simulink model "43_BusNetworkElectricityTransmissionModel"  (R2023b)
settings: Solver=VariableStepAuto  StartTime=0.0  StopTime=0.8  RelTol=1e-3
model workspace (MAT data in the model file):
  BESS_Fp_KDroop = 0.025
  BESS_KSI = 817
  BESS_PWM_fs = 560
  BESS_P_Ki = 0.5
  BESS_P_Kp = 0.0636
  BESS_Pnom = 3000000
  BESS_Q_Ki = 1
  BESS_Q_Kp = 0.0257
  BESS_Vd_Ki = 850
  BESS_Vd_Kp = 0.216
  BESS_Vnom = 1000
  BESS_Vq_KDroop = 0.025
  BESS_Vq_Ki = 850
  BESS_Vq_Kp = 0.216
  Compensation_Ki = 30
  Compensation_Kp = 3
  DC_Ki = 400
  DC_Kp = 8
  F = 0.01
  Flux_min = 0.5
  Grid_Freq_PWM = 2700
  Grid_Ireg_Ki = 5
  Grid_Ireg_Kp = 0.83
  Grid_Ireg_lim = 1.1
  Grid_Modindex_Upper = 1.1
  Grid_conv_Imax = 0.8
  H = 0.685
  Idref_max = 0.9
  Iqref_Tc = 0.3
  Ki_Var = 0.05
  Ki_Vreg = 20
  Ksh = 1.1
  L_pu = 0.3
  Llr = 0.16
  Lls = 0.18
  Lm = 2.9
  LowLoad_P = 130
  Nb_wt = 6
  P_mech = 1080000
  PeakShav_P = 200
  Pitch_Ki = 0
  Pitch_Kp = 150
  Pitch_Max = 27
  Pitch_Tc = 0.01
  Pitch_rate = 10
  Q_Filt = 50
  R_pu = 0.003
  Rotor_Freq_PWM = 1620
  Rotor_Ireg_Ki = 8
  Rotor_Ireg_Kp = 0.6
  Rotor_Ireg_lim = 0.1
  Rotor_Modindex_Upper = 2
  Rr = 0.016
  Rs = 0.023
  SOCBESS : Simulink.Parameter (value not decoded)
  T_set = 0.0001
  Tp = 5e-05
  Ts = 5e-06
  Var_C_Filt = 720000
  Var_reg_max = 1.1
  Var_reg_min = 0.9
  WT_Coeff = [0.645 116 0.4 5 21 0.00912 0.08 0.035]
  WT_H = 4.32
  WT_IGBTRon = 5.931
  WT_Param = [91.204 10143]
  Wind_Freq_Filt = 10000
  Wind_Freq_nom = 60
  Wind_P_nom = 1200000
  Wind_Rotor_V_nom = 1950
  Wind_V_nom = 500
  Zeta_Filt = 0.707106781187
  init = [-0.2 0 0 0 0 0 0 0]
  p = 3
  torque0 = 0.83
  v_Ki = 0.1
  v_Kp = 3.6
  v_Max = 1.2
  v_Min = 0.7
  v_T = 5
  vreg_max = 1
  wind_VDC_nom = 1150
  wt0 = 1.2
undefined symbols (not defined in the file): D1, D11, Delta, DiscIntNeverNeededParam, Iabc, Ion, Lithium, P, Q, Vabc
libraries: powerlib_extras x156, spsSeriesRLCBranchLib x66, spsLoadFlowBusLib x43, spsThreePhaseSeriesRLCLoadLib x33, spsThreePhaseTransformerTwoWindingsLib x32, spsThreePhaseVIMeasurementLib x30, simulink_extras x30, spsDistributedParametersLineLib x22, spsGenericPowerSystemStabilizerLib x20, spsSynchronousMachinepuStandardLib x10, spsExcitationSystemLib x10, spsHydraulicTurbineandGovernorLib x10
(part 8 of 19)

== system 43_BusNetworkElectricityTransmissionModel/400 kV Solar Farm/VSC Control/Uabc_ref Generation max (m) = 1 ==
  note: (Correction for transformer
      |  D1 connection)
  note: (Correction for delai of Ts_Control)
  wt : Inport
  VdVq_conv : Inport  Port=2
  Add1 : Sum  Inputs=++++
  Add2 : Sum
  Complex to Magnitude-Angle : ComplexToMagnitudeAngle
  Constant : Constant  Value=-pi/6
  Constant1 : Constant  Value=Vnom_dc
  Constant2 : Constant  Value="[ 0  -2*pi/3  2*pi/3  ]"
  Constant3 : Constant  Value=Vnom_sec*sqrt(2)/sqrt(3)
  Constant4 : Constant  Value=Ts*Fnom*(2*pi)
  Demux1 : Demux  Outputs=2
  Gain1 : Gain  Gain=1/2
  Product : Product  Inputs=*/  RndMeth=Zero
  Product1 : Product  Inputs=*/  RndMeth=Zero
  Product2 : Product  Inputs=**  RndMeth=Zero
  Real-Imag to Complex : RealImagToComplex
  Saturation : Saturate  UpperLimit=1  LowerLimit=0
  Trigonometric Function : Trigonometry
  Uabc_ref : Outport  VectorParamsAs1DForOutWhenUnconnected=off
  wires:
  Complex to Magnitude-Angle/1 -> Saturation/1
  Constant1/1 -> Gain1/1
  VdVq_conv/1 -> Product1/1
  Product1/1 -> Demux1/1
  Gain1/1 -> Product/1
  Real-Imag to Complex/1 -> Complex to Magnitude-Angle/1
  Demux1/1 -> Real-Imag to Complex/1
  Demux1/2 -> Real-Imag to Complex/2
  Constant2/1 -> Add1/2
  Constant/1 -> Add1/3
  Constant3/1 -> Product/2
  Product/1 -> Product1/2
  Complex to Magnitude-Angle/2 -> Add2/1
  Add1/1 -> Add2/2
  Add2/1 -> Trigonometric Function/1
  Saturation/1 -> Product2/1
  Trigonometric Function/1 -> Product2/2
  Product2/1 -> Uabc_ref/1
  wt/1 -> Add1/1
  Constant4/1 -> Add1/4

== system 43_BusNetworkElectricityTransmissionModel/400 kV Solar Farm/VSC Control/VDC Regulator ==
  Vdc_mes : Inport  PortDimensions=1
  Vdc_ref : Inport  Port=2  PortDimensions=1
  PI : slpidlib/PID Controller  Controller=PI  Form=Parallel  TimeDomain=Discrete-time  UseExternalTs=off  SampleTime=Ts  IntegratorMethod=Trapezoidal  FilterMethod=Forward Euler  ControllerParametersSource=internal  P=Kp_VDCreg  I=Ki_VDCreg  UseKiTs=off  D=0  N=100  UseFilter=on  TunerSelectOption=Transfer Function Based (PID Tuner App)  InitialConditionSource=internal  InitialConditionForIntegrator=0  InitialConditionForFilter=0  DifferentiatorICPrevScaledInput=0  ExternalReset=none  TrackingMode=off  Kt=1  LimitOutput=on  SatLimitsSource=internal  UpperSaturationLimit=1.5  LowerSaturationLimit=-1.5  LinearizeAsGain=off  AntiWindupMode=none  Kb=1  LimitIntegrator=off  UpperIntegratorSaturationLimit=inf  LowerIntegratorSaturationLimit=-inf  POutMin=[]  POutMax=[]  IOutMin=[]  IOutMax=[]  DOutMin=[]  DOutMax=[]  NOutMin=[]  NOutMax=[]  SumOutMin=[]  SumOutMax=[]  SaturationOutMin=[]  SaturationOutMax=[]  PParamMin=[]  PParamMax=[]  IParamMin=[]  IParamMax=[]  DParamMin=[]  DParamMax=[]  NParamMin=[]  NParamMax=[]  KbParamMin=[]  KbParamMax=[]  KtParamMin=[]  KtParamMax=[]  KbOutMin=[]  KbOutMax=[]  KtOutMin=[]  KtOutMax=[]  IntegratorOutMin=[]  IntegratorOutMax=[]  FilterOutMin=[]  FilterOutMax=[]  SumI1OutMin=[]  SumI1OutMax=[]  SumI2OutMin=[]  SumI2OutMax=[]  SumI3OutMin=[]  SumI3OutMax=[]  SumI4OutMin=[]  SumI4OutMax=[]  SumDOutMin=[]  SumDOutMax=[]  DifferentiatorOutMin=[]  DifferentiatorOutMax=[]  FilterDiffOutCoefMin=[]  FilterDiffOutCoefMax=[]  ReciprocalOutMin=[]  ReciprocalOutMax=[]  SumDenOutMin=[]  SumDenOutMax=[]  SumNumOutMin=[]  SumNumOutMax=[]  DivideOutMin=[]  DivideOutMax=[]  UdiffTsProdOutMin=[]  UdiffTsProdOutMax=[]  NTsProdOutMin=[]  NTsProdOutMax=[]  UintegralTsProdOutMin=[]  UintegralTsProdOutMax=[]  UngainTsProdOutMin=[]  UngainTsProdOutMax=[]  ClampingZeroOutDataTypeStr=Inherit: Inherit via back propagation  ClampingZeroOutMin=[]  ClampingZeroOutMax=[]  FilterDenConstantOutDataTypeStr=Inherit: Inherit via back propagation  FilterDenConstantOutMin=[]  FilterDenConstantOutMax=[]  PCopyOutDataTypeStr=Inherit: Inherit via back propagation  PCopyOutMin=[]  PCopyOutMax=[]  NCopyOutDataTypeStr=Inherit: Inherit via back propagation  NCopyOutMin=[]  NCopyOutMax=[]  IntegratorContinuousStateAttributes=''  IntegratorStateMustResolveToSignalObject=off  IntegratorRTWStateStorageClass=Auto  FilterContinuousStateAttributes=''  FilterStateMustResolveToSignalObject=off  FilterRTWStateStorageClass=Auto  ParallelPVariant=InternalParameters  IdealPVariant=Disabled  IVariant=InternalParameters  DVariant=Disabled  IntegratorVariant=Discrete  SatVariant=Enabled  AWVariant=Passthrough  PCopyVariant=Disabled  TRVariant=Disabled  FdbkBlocksVariant=Forward  IdealPFdbkVariant=Disabled  SatFdbkVariant=Disabled  DerivativeFilterVariant=Disabled  NVariant=Disabled  NCopyVariant=Disabled_SignalSpec  FilterICVariant=Disabled  IntegratorICVariant=InternalICs  ExternalResetVariant=Disabled  TRSumVariant=Passthrough  SumFdbkVariant=Disabled  SumVariant=Sum_PI  TsampFilterVariant=InternalTs  TsampNgainVariant=Passthrough  TsampIntegralVariant=Disabled_SignalSpec  ExternalSaturationOutDataTypeStr=Inherit: Same as second input
  Rtot_pu3 : Gain  Gain=1/Vnom_dc  SaturateOnIntegerOverflow=on  OutDataTypeStr=Inherit: Same as input  ParamDataTypeStr=Inherit: Same as input
  Sum : Sum  Inputs=|+-
  Id_ref : Outport  SampleTime=Ts  InitialOutput=0  VectorParamsAs1DForOutWhenUnconnected=off
  wires:
  Sum/1 -> Rtot_pu3/1
  Vdc_mes/1 -> Sum/1
  Vdc_ref/1 -> Sum/2
  Rtot_pu3/1 -> PI/1
  PI/1 -> Id_ref/1

== system 43_BusNetworkElectricityTransmissionModel/Li-ion BESS/BESS/BESS and Controller ==
  Control : Inport
  Grid_Data : Inport  Port=2
  BESS : Subsystem
      settings: PortSchema="{\"entries\":[{\"content\":{\"sides\":[{\"content\":{\"connectorIds\":[\"In1\",\"LConn1\",\"LConn2\",\"LConn3\"]},\"type\":\"ConnectorPlacement.EquallySpacedRectSide\",\"uuid\":\"a1d953a5-733c-426a-ade3-c5bdc4580032\"},{\"content\":{\"connectorIds\":[\"In2\",\"Out1\"],\"side\":\"RIGHT\"},\"type\":\"ConnectorPlacement.EquallySpacedRectSide\",\"uuid\":\"97f93640-474b-46b7-9c6f-aa155152508d\"},{\"content\":{\"side\":\"TOP\"},\"type\":\"ConnectorPlacement.EquallySpacedRectSide\",\"uuid\":\"f50f5af6-db0c-4ef7-bd71-a55c9ecceb9a\"}]},\"type\":\"ConnectorPlacement.EquallySpacedConnector\",\"uuid\":\"22d19704-c3d4-4f3f-ab22-c7739cf2dc05\"}],\"packageUris\":[\"http://schema.mathworks.com/mf0/Connector/R2020b\"],\"version\":\"1.0\"}"
  BESS Control : Subsystem
      settings: PortSchema="{\"entries\":[{\"content\":{\"sides\":[{\"content\":{\"connectorIds\":[\"In1\",\"In2\",\"In3\"]},\"type\":\"ConnectorPlacement.EquallySpacedRectSide\",\"uuid\":\"c98aaab3-ca22-4a29-92cf-a6c6fcb60087\"},{\"content\":{\"connectorIds\":[\"Out1\",\"Out2\",\"Out3\"],\"side\":\"RIGHT\"},\"type\":\"ConnectorPlacement.EquallySpacedRectSide\",\"uuid\":\"d7f3f6ce-ab70-4311-9ddf-7d43df8329f4\"},{\"content\":{\"connectorIds\":[\"In4\"],\"side\":\"TOP\"},\"type\":\"ConnectorPlacement.EquallySpacedRectSide\",\"uuid\":\"f981cd0b-01ce-44ec-8804-34a9753b0161\"}]},\"type\":\"ConnectorPlacement.EquallySpacedConnector\",\"uuid\":\"874b0b3a-e878-43a5-a035-a40a954e1edd\"}],\"packageUris\":[\"http://schema.mathworks.com/mf0/Connector/R2020b\"],\"version\":\"1.0\"}"
  BMS : Subsystem
      settings: PortSchema="{\"entries\":[{\"content\":{\"sides\":[{\"content\":{\"connectorIds\":[\"In1\",\"Out2\",\"Out3\"]},\"type\":\"ConnectorPlacement.EquallySpacedRectSide\",\"uuid\":\"90a0640c-776d-46b7-b062-0b224e57e494\"},{\"content\":{\"connectorIds\":[\"Out1\",\"In3\"],\"side\":\"RIGHT\"},\"type\":\"ConnectorPlacement.EquallySpacedRectSide\",\"uuid\":\"dd2d8a9e-5ca6-4aee-a7d3-a7e9cd622cb5\"},{\"content\":{\"connectorIds\":[\"In2\"],\"side\":\"TOP\"},\"type\":\"ConnectorPlacement.EquallySpacedRectSide\",\"uuid\":\"90e91986-9fe4-4870-9173-40c6af706bc8\"}]},\"type\":\"ConnectorPlacement.EquallySpacedConnector\",\"uuid\":\"b96376bb-fdeb-4c13-a438-fbd280210e00\"}],\"packageUris\":[\"http://schema.mathworks.com/mf0/Connector/R2020b\"],\"version\":\"1.0\"}"
  Bus Creator : BusCreator  Inputs=4
  Bus Creator1 : BusCreator  Inputs=2
  Inverter Measurement : Subsystem
  Three-Phase Series RLC Branch : spsThreePhaseSeriesRLCBranchLib/Three-Phase Series RLC Branch  LConnTagsString=A|B|C  RConnTagsString=A|B|C  BranchType=RL  Resistance=1e-1  Inductance=1e-2  Capacitance=1e-6  Measurements=None
  Three-Phase Series RLC Load : spsThreePhaseSeriesRLCLoadLib/Three-Phase Series RLC Load  LConnTagsString=A|B|C  Configuration=Y (grounded)  NominalVoltage=1000  Vabc=[1e3 1e3 1e3]  Vabcp=[1e3 1e3 1e3]  NominalFrequency=60  UnbalancedPower=off  ActivePower=155346  InductivePower=0  CapacitivePower=1e6  Pabc=[10e3 9e3 11e3]  QLabc=[100 90 110]  QCabc=[100 90 110]  Pabcp=[10e3 9e3 11e3]  QLabcp=[100 90 110]  QCabcp=[100 90 110]  Measurements=None  LoadType=constant Z
  Three-Phase Breaker : spsThreePhaseBreakerLib/Three-Phase Breaker  InitialState=open  SwitchA=on  SwitchB=on  SwitchC=on  SwitchTimes="[0  3]"  External=off  BreakerResistance=0.01  SnubberResistance=1e6  SnubberCapacitance=inf  Measurements=None
  A : PMIOPort  Side=Left
  B : PMIOPort  Port=2  Side=Left
  C : PMIOPort  Port=3  Side=Left
  BESS_Data : Outport
  wires:
  Control/1 -> BMS/2(Control), BESS Control/4(Control)
  BMS/2(Stat_BESS) -> Bus Creator/2
  BMS/3(Stat_SOC) -> Bus Creator/3
  Inverter Measurement/1(BESS_Data) -> BESS Control/3(BESS_Data), Bus Creator1/1  "BESS_Data2"
  BESS/1(SOC) -> Bus Creator/4, BMS/3(SOC)  "SoC"
  [BESS_Command] -> Bus Creator/1, BMS/1(BESS_Command)
  Grid_Data/1 -> BESS Control/2(Grid_Data)
  BESS Control/3(BESS_Control) -> Bus Creator1/2  "BMS_Data"
  Bus Creator1/1 -> BESS_Data/1
  BESS Control/2(BMS) -> [BESS_Command]
  BESS Control/1(PWM_Wave) -> BESS/1(PWM wave)
  Bus Creator/1 -> BESS Control/1(BMS_BESS)
  BMS/1(Gate_Op) -> BESS/2(Gate_Op)
  connections:
  Three-Phase Series RLC Branch/RConn3 -- Inverter Measurement/LConn3 -- Three-Phase Series RLC Load/LConn3
  Three-Phase Series RLC Load/LConn1 -- Three-Phase Series RLC Branch/RConn1 -- Inverter Measurement/LConn1
  Three-Phase Series RLC Branch/RConn2 -- Three-Phase Series RLC Load/LConn2 -- Inverter Measurement/LConn2
  Inverter Measurement/RConn1 -- Three-Phase Breaker/LConn1
  Three-Phase Breaker/LConn2 -- Inverter Measurement/RConn2
  Inverter Measurement/RConn3 -- Three-Phase Breaker/LConn3
  Three-Phase Breaker/RConn1 -- A/RConn1
  B/RConn1 -- Three-Phase Breaker/RConn2
  Three-Phase Breaker/RConn3 -- C/RConn1
  BESS/LConn1 -- Three-Phase Series RLC Branch/LConn1
  BESS/LConn2 -- Three-Phase Series RLC Branch/LConn2
  BESS/LConn3 -- Three-Phase Series RLC Branch/LConn3

== system 43_BusNetworkElectricityTransmissionModel/Li-ion BESS/BESS/Grid Measurement ==
  Bus Creator : BusCreator  Inputs=Vabc,Iabc,P,Q
  Power Calculation : Subsystem
  Scope : Scope  NumInputPorts=2
  Three-Phase V-I Measurement : spsThreePhaseVIMeasurementLib/Three-Phase V-I Measurement  VoltageMeasurement=phase-to-ground  SetLabelV=off  LabelV=BESS_Vabc  Vpu=off  VpuLL=off  CurrentMeasurement=yes  SetLabelI=off  LabelI=Iabc  Ipu=off  Pbase=100e6  Vbase=500e3  OutputType=Complex  PhasorSimulation=off  PSBequivalent=0
  A : PMIOPort  Side=Left
  B : PMIOPort  Port=2  Side=Left
  C : PMIOPort  Port=3  Side=Left
  A1 : PMIOPort  Port=4  Side=Right
  B1 : PMIOPort  Port=5  Side=Right
  C1 : PMIOPort  Port=6  Side=Right
  Grid : Outport
  wires:
  Three-Phase V-I Measurement/1 -> Bus Creator/1, Power Calculation/1(Vabc)  "Vabc"
  Three-Phase V-I Measurement/2 -> Bus Creator/2, Power Calculation/2(Iabc)  "Iabc"
  Power Calculation/2(Q) -> Scope/2, Bus Creator/4  "Q"
  Bus Creator/1 -> Grid/1
  Power Calculation/1(P) -> Scope/1, Bus Creator/3  "P"
  connections:
  Three-Phase V-I Measurement/RConn2 -- B1/RConn1
  Three-Phase V-I Measurement/LConn2 -- B/RConn1
  Three-Phase V-I Measurement/LConn3 -- C/RConn1
  C1/RConn1 -- Three-Phase V-I Measurement/RConn3
  A1/RConn1 -- Three-Phase V-I Measurement/RConn1
  A/RConn1 -- Three-Phase V-I Measurement/LConn1

== system 43_BusNetworkElectricityTransmissionModel/Li-ion BESS/Control/Monitoring and measurement  ==
  BESS_Data : Inport
  AND : Logic  IconShape=distinctive  AllPortsSameDT=off  OutDataTypeStr=boolean
  AND1 : Logic  IconShape=distinctive  AllPortsSameDT=off  OutDataTypeStr=boolean
  BESS Measurements : Subsystem
  BESS_Data1 : InportShadow
  BESS_Data3 : InportShadow
  Bus Selector : BusSelector  OutputSignals=Grid_Data.Vabc,Grid_Data.Iabc
  Bus Selector1 : BusSelector  OutputSignals=BESS.BMS_Data.Stat_SOC,BESS.BMS_Data.SoC.MAXSOC,BESS.BMS_Data.SoC.MINSOC,BESS.BMS_Data.signal1.BESS_Charging,BESS.BMS_Data.Stat_BESS,BESS.BMS_Data.signal1.BESS_Discharging
  Bus Selector3 : BusSelector  OutputSignals=BESS.BESS_Data2.P,BESS.BESS_Data2.Q,BESS.BESS_Data2.Vabc,BESS.BESS_Data2.Iabc
  Subsystem : Subsystem
      settings: PortSchema="{\"entries\":[{\"content\":{\"sides\":[{\"content\":{\"connectorIds\":[]},\"type\":\"ConnectorPlacement.EquallySpacedRectSide\",\"uuid\":\"1c641b2f-4abd-4026-9424-76979de06f8f\"},{\"content\":{\"connectorIds\":[\"Out1\"],\"side\":\"RIGHT\"},\"type\":\"ConnectorPlacement.EquallySpacedRectSide\",\"uuid\":\"ecc6cae9-a0ed-4b97-bfc8-2766ee0a977d\"},{\"content\":{\"connectorIds\":[],\"side\":\"TOP\"},\"type\":\"ConnectorPlacement.EquallySpacedRectSide\",\"uuid\":\"9585e64e-ef0f-4765-963d-d981a90f0760\"},{\"content\":{\"connectorIds\":[\"In1\"],\"side\":\"BOTTOM\"},\"type\":\"ConnectorPlacement.EquallySpacedRectSide\",\"uuid\":\"12697e63-83ff-496d-a295-b3930fbd5601\"}]},\"type\":\"ConnectorPlacement.EquallySpacedConnector\",\"uuid\":\"b5fa0ee0-8f2a-44ad-b4f1-35d45efa1097\"}],\"packageUris\":[\"http://schema.mathworks.com/mf0/Connector/R2020b\"],\"version\":\"1.0\"}"
  Subsystem1 : Subsystem
      settings: PortSchema="{\"entries\":[{\"content\":{\"sides\":[{\"content\":{\"connectorIds\":[]},\"type\":\"ConnectorPlacement.EquallySpacedRectSide\",\"uuid\":\"1c641b2f-4abd-4026-9424-76979de06f8f\"},{\"content\":{\"connectorIds\":[\"Out1\"],\"side\":\"RIGHT\"},\"type\":\"ConnectorPlacement.EquallySpacedRectSide\",\"uuid\":\"ecc6cae9-a0ed-4b97-bfc8-2766ee0a977d\"},{\"content\":{\"connectorIds\":[\"In1\"],\"side\":\"TOP\"},\"type\":\"ConnectorPlacement.EquallySpacedRectSide\",\"uuid\":\"9585e64e-ef0f-4765-963d-d981a90f0760\"},{\"content\":{\"connectorIds\":[],\"side\":\"BOTTOM\"},\"type\":\"ConnectorPlacement.EquallySpacedRectSide\",\"uuid\":\"12697e63-83ff-496d-a295-b3930fbd5601\"}]},\"type\":\"ConnectorPlacement.EquallySpacedConnector\",\"uuid\":\"b5fa0ee0-8f2a-44ad-b4f1-35d45efa1097\"}],\"packageUris\":[\"http://schema.mathworks.com/mf0/Connector/R2020b\"],\"version\":\"1.0\"}"
  THD : Scope  NumInputPorts=2
  Total Harmonic Distortion2 : eeTotalHarmonicDistorsion/Total Harmonic Distortion  f=60  Ts=Ts
      settings: LibrarySourceBlock=|
      | ee_sl_lib/Measurements/Total Harmonic
      | Distortion
  Total Harmonic Distortion3 : eeTotalHarmonicDistorsion/Total Harmonic Distortion  f=60  Ts=Ts
      settings: LibrarySourceBlock=|
      | ee_sl_lib/Measurements/Total Harmonic
      | Distortion
  tag scope: BESS_Charge_Actual=global, BESS_Charging_Com=global, BESS_Discharge_Actual=global, BESS_Discharging_Com=global, BESS_MAXSOC=global, BESS_MINSOC=global, BESS_SOC=global, Stat_BESS=global
  wires:
  Bus Selector3/1 -> BESS Measurements/1(BESS_P)  "<P>"
  Bus Selector1/5 -> [Stat_BESS], Subsystem/1(mBESS), Subsystem1/1(mBESS)  "<Stat_BESS>"
  Bus Selector1/6 -> [BESS_Discharging_Com], AND/1  "<BESS_Discharging>"
  Bus Selector1/2 -> [BESS_MAXSOC]  "<MAXSOC>"
  Bus Selector1/3 -> [BESS_MINSOC]  "<MINSOC>"
  Bus Selector1/1 -> [BESS_SOC]  "<Stat_SOC>"
  AND/1 -> [BESS_Discharge_Actual]  "BESS Discharge"
  Bus Selector1/4 -> [BESS_Charging_Com], AND1/2  "<BESS_Charging>"
  AND1/1 -> [BESS_Charge_Actual]  "BESS Charge"
  Subsystem/1(Out1) -> AND/2
  Subsystem1/1(Out1) -> AND1/1
  Total Harmonic Distortion2/1 -> THD/1  "Grid Voltage THD (%)"
  Total Harmonic Distortion3/1 -> THD/2  "Grid Current THD (%)"
  Bus Selector/2 -> Total Harmonic Distortion3/1  "<Iabc>"
  BESS_Data/1 -> Bus Selector/1
  Bus Selector/1 -> Total Harmonic Distortion2/1  "<Vabc>"
  BESS_Data1/1 -> Bus Selector1/1
  BESS_Data3/1 -> Bus Selector3/1
  Bus Selector3/2 -> BESS Measurements/2(BESS_Q)  "<Q>"
  Bus Selector3/3 -> BESS Measurements/3(BESS Voltage)  "<Vabc>"
  Bus Selector3/4 -> BESS Measurements/4(BESS Current)  "<Iabc>"

== system 43_BusNetworkElectricityTransmissionModel/North Network/Regulators 7/Turbine and Excitation Regulators ==
  pref : Inport
  w : Inport  Port=2
  Pe 0 : Inport  Port=3
  Vref : Inport  Port=4
  Vm : Inport  Port=5
  Add : Sum  Inputs=+-
  Complex to Real-Imag : ComplexToRealImag
  Excitation System : spsExcitationSystemLib/Excitation System  tr=20e-3  reg=[ 300, 0.001 ]  exc=[ 1, 0 ]  tgr=[ 0, 0 ]  damp=[ 0.001, 0.1 ]  sat=[ 0, 0 ]  lim=[ -11.5, 11.5, 0 ]  v0="[1.0  1.28]"
      settings: LibrarySourceBlock=sps_lib/Electrical Machines/Synchronous Machine Control/Excitation System
  Hydraulic Turbine and Governor : spsHydraulicTurbineandGovernorLib/Hydraulic Turbine and Governor  sm="[ 10/3  0.07 ]"  gate="[  0.01  0.97518  -0.1  0.1 ]"  reg="[  0.05  1.163  0.105  0  0.01  ]"  hyd="[  0  2.67  ]"  dref=0  po=0.7516
      settings: LibrarySourceBlock=|
      | sps_lib/Electrical Machines/Synchronous Machine Control/Hydraulic Turbine
      | and Governor
  Stabilitator : Subsystem
  Terminator : Terminator
  wref : Constant
  wref1 : Constant
  Pm : Outport
  Vf : Outport  Port=2
  wires:
  pref/1 -> Hydraulic Turbine and Governor/2
  Complex to Real-Imag/2 -> Excitation System/3
  wref/1 -> Hydraulic Turbine and Governor/1
  Add/1 -> Stabilitator/3(dw), Hydraulic Turbine and Governor/5
  Vm/1 -> Complex to Real-Imag/1
  Pe 0/1 -> Stabilitator/2(Pe), Hydraulic Turbine and Governor/4
  Hydraulic Turbine and Governor/2 -> Terminator/1
  Stabilitator/1(Out1) -> Excitation System/4
  w/1 -> Add/1, Hydraulic Turbine and Governor/3
  Excitation System/1 -> Vf/1
  Hydraulic Turbine and Governor/1 -> Pm/1, Stabilitator/1(Pm)
  Vref/1 -> Excitation System/1
  wref1/1 -> Add/2
  Complex to Real-Imag/1 -> Excitation System/2

== system 43_BusNetworkElectricityTransmissionModel/North Network/Regulators 8/Turbine and Excitation Regulators ==
  pref : Inport
  w : Inport  Port=2
  Pe 0 : Inport  Port=3
  Vref : Inport  Port=4
  Vm : Inport  Port=5
  Add : Sum  Inputs=+-
  Complex to Real-Imag : ComplexToRealImag
  Excitation System : spsExcitationSystemLib/Excitation System  tr=20e-3  reg=[ 300, 0.001 ]  exc=[ 1, 0 ]  tgr=[ 0, 0 ]  damp=[ 0.001, 0.1 ]  sat=[ 0, 0 ]  lim=[ -11.5, 11.5, 0 ]  v0="[1.0  1.28]"
      settings: LibrarySourceBlock=sps_lib/Electrical Machines/Synchronous Machine Control/Excitation System
  Hydraulic Turbine and Governor : spsHydraulicTurbineandGovernorLib/Hydraulic Turbine and Governor  sm="[ 10/3  0.07 ]"  gate="[  0.01  0.97518  -0.1  0.1 ]"  reg="[  0.05  1.163  0.105  0  0.01  ]"  hyd="[  0  2.67  ]"  dref=0  po=0.7516
      settings: LibrarySourceBlock=|
      | sps_lib/Electrical Machines/Synchronous Machine Control/Hydraulic Turbine
      | and Governor
  Stabilitator : Subsystem
  Terminator : Terminator
  wref : Constant
  wref1 : Constant
  Pm : Outport
  Vf : Outport  Port=2
  wires:
  pref/1 -> Hydraulic Turbine and Governor/2
  Complex to Real-Imag/2 -> Excitation System/3
  wref/1 -> Hydraulic Turbine and Governor/1
  Add/1 -> Stabilitator/3(dw), Hydraulic Turbine and Governor/5
  Vm/1 -> Complex to Real-Imag/1
  Pe 0/1 -> Stabilitator/2(Pe), Hydraulic Turbine and Governor/4
  Hydraulic Turbine and Governor/2 -> Terminator/1
  Stabilitator/1(Out1) -> Excitation System/4
  w/1 -> Add/1, Hydraulic Turbine and Governor/3
  Excitation System/1 -> Vf/1
  Hydraulic Turbine and Governor/1 -> Pm/1, Stabilitator/1(Pm)
  Vref/1 -> Excitation System/1
  wref1/1 -> Add/2
  Complex to Real-Imag/1 -> Excitation System/2

== system 43_BusNetworkElectricityTransmissionModel/North Network/Regulators 9/Turbine and Excitation Regulators ==
  pref : Inport
  w : Inport  Port=2
  Pe 0 : Inport  Port=3
  Vref : Inport  Port=4
  Vm : Inport  Port=5
  Add : Sum  Inputs=+-
  Complex to Real-Imag : ComplexToRealImag
  Excitation System : spsExcitationSystemLib/Excitation System  tr=20e-3  reg=[ 300, 0.001 ]  exc=[ 1, 0 ]  tgr=[ 0, 0 ]  damp=[ 0.001, 0.1 ]  sat=[ 0, 0 ]  lim=[ -11.5, 11.5, 0 ]  v0="[1.0  1.28]"
      settings: LibrarySourceBlock=sps_lib/Electrical Machines/Synchronous Machine Control/Excitation System
  Hydraulic Turbine and Governor : spsHydraulicTurbineandGovernorLib/Hydraulic Turbine and Governor  sm="[ 10/3  0.07 ]"  gate="[  0.01  0.97518  -0.1  0.1 ]"  reg="[  0.05  1.163  0.105  0  0.01  ]"  hyd="[  0  2.67  ]"  dref=0  po=0.7516
      settings: LibrarySourceBlock=|
      | sps_lib/Electrical Machines/Synchronous Machine Control/Hydraulic Turbine
      | and Governor
  Stabilitator : Subsystem
  Terminator : Terminator
  wref : Constant
  wref1 : Constant
  Pm : Outport
  Vf : Outport  Port=2
  wires:
  pref/1 -> Hydraulic Turbine and Governor/2
  Complex to Real-Imag/2 -> Excitation System/3
  wref/1 -> Hydraulic Turbine and Governor/1
  Add/1 -> Stabilitator/3(dw), Hydraulic Turbine and Governor/5
  Vm/1 -> Complex to Real-Imag/1
  Pe 0/1 -> Stabilitator/2(Pe), Hydraulic Turbine and Governor/4
  Hydraulic Turbine and Governor/2 -> Terminator/1
  Stabilitator/1(Stab) -> Excitation System/4
  w/1 -> Add/1, Hydraulic Turbine and Governor/3
  Excitation System/1 -> Vf/1
  Hydraulic Turbine and Governor/1 -> Pm/1, Stabilitator/1(Pm)
  Vref/1 -> Excitation System/1
  wref1/1 -> Add/2
  Complex to Real-Imag/1 -> Excitation System/2

== system 43_BusNetworkElectricityTransmissionModel/Regulators 10/Turbine and Excitation Regulators/Stabilitator ==
  Pm : Inport
  Pe : Inport  Port=2
  dw : Inport  Port=3
  Add1 : Sum  Inputs=+-
  Generic Power System Stabilizer : spsGenericPowerSystemStabilizerLib/Generic Power System Stabilizer  Tsensor=30e-3  K=20  Twashout=2  Tleadlag1=[50e-3 20e-3]  Tleadlag2=[3 5.4]  VSlimits=[-0.15 0.15]  Vinit=0  Plot_On=off  MagdB_On=on  FreqRange=logspace(-2,2,500)
      settings: LibrarySourceBlock=|
      | sps_lib/Electrical Machines/Synchronous Machine Control/Generic
      | Power System Stabilizer
  Generic Power System Stabilizer1 : spsGenericPowerSystemStabilizerLib/Generic Power System Stabilizer  Tsensor=30e-3  K=20  Twashout=2  Tleadlag1=[50e-3 20e-3]  Tleadlag2=[3 5.4]  VSlimits=[-0.15 0.15]  Vinit=0  Plot_On=off  MagdB_On=on  FreqRange=logspace(-2,2,500)
      settings: LibrarySourceBlock=|
      | sps_lib/Electrical Machines/Synchronous Machine Control/Generic
      | Power System Stabilizer
  Ground : Ground
  Multiport Switch : MultiPortSwitch  DiagnosticForDefault=None  SaturateOnIntegerOverflow=off  InputSameDT=off
  Out1 : Outport
  wires:
  Pm/1 -> Add1/1
  Generic Power System Stabilizer1/1 -> Multiport Switch/4
  Pe/1 -> Add1/2
  Add1/1 -> Generic Power System Stabilizer/1
  Generic Power System Stabilizer/1 -> Multiport Switch/3
  dw/1 -> Generic Power System Stabilizer1/1
  Ground/1 -> Multiport Switch/2
  [PSS_modes] -> Multiport Switch/1
  Multiport Switch/1 -> Out1/1

== system 43_BusNetworkElectricityTransmissionModel/South Network/Regulators 1/Turbine and Excitation Regulators ==
  pref : Inport
  w : Inport  Port=2
  Pe 0 : Inport  Port=3
  Vref : Inport  Port=4
  Vm : Inport  Port=5
  Add : Sum  Inputs=+-
  Complex to Real-Imag : ComplexToRealImag
  Excitation System : spsExcitationSystemLib/Excitation System  tr=20e-3  reg=[ 300, 0.001 ]  exc=[ 1, 0 ]  tgr=[ 0, 0 ]  damp=[ 0.001, 0.1 ]  sat=[ 0, 0 ]  lim=[ -11.5, 11.5, 0 ]  v0="[1.0  1.28]"
      settings: LibrarySourceBlock=sps_lib/Electrical Machines/Synchronous Machine Control/Excitation System
  Hydraulic Turbine and Governor : spsHydraulicTurbineandGovernorLib/Hydraulic Turbine and Governor  sm="[ 10/3  0.07 ]"  gate="[  0.01  0.97518  -0.1  0.1 ]"  reg="[  0.05  1.163  0.105  0  0.01  ]"  hyd="[  0  2.67  ]"  dref=0  po=0.7516
      settings: LibrarySourceBlock=|
      | sps_lib/Electrical Machines/Synchronous Machine Control/Hydraulic Turbine
      | and Governor
  Stabilitator : Subsystem
  Terminator : Terminator
  wref : Constant
  wref1 : Constant
  Pm : Outport
  Vf : Outport  Port=2
  wires:
  pref/1 -> Hydraulic Turbine and Governor/2
  Complex to Real-Imag/2 -> Excitation System/3
  wref/1 -> Hydraulic Turbine and Governor/1
  Add/1 -> Stabilitator/3(dw), Hydraulic Turbine and Governor/5
  Vm/1 -> Complex to Real-Imag/1
  Pe 0/1 -> Stabilitator/2(Pe), Hydraulic Turbine and Governor/4
  Hydraulic Turbine and Governor/2 -> Terminator/1
  Stabilitator/1(Out1) -> Excitation System/4
  w/1 -> Add/1, Hydraulic Turbine and Governor/3
  Excitation System/1 -> Vf/1
  Hydraulic Turbine and Governor/1 -> Pm/1, Stabilitator/1(Pm)
  Vref/1 -> Excitation System/1
  wref1/1 -> Add/2
  Complex to Real-Imag/1 -> Excitation System/2

== system 43_BusNetworkElectricityTransmissionModel/South Network/Regulators 2/Turbine and Excitation Regulators ==
  pref : Inport
  w : Inport  Port=2
  Pe 0 : Inport  Port=3
  Vref : Inport  Port=4
  Vm : Inport  Port=5
  Add : Sum  Inputs=+-
  Complex to Real-Imag : ComplexToRealImag
  Excitation System : spsExcitationSystemLib/Excitation System  tr=20e-3  reg=[ 300, 0.001 ]  exc=[ 1, 0 ]  tgr=[ 0, 0 ]  damp=[ 0.001, 0.1 ]  sat=[ 0, 0 ]  lim=[ -11.5, 11.5, 0 ]  v0="[1.0  1.28]"
      settings: LibrarySourceBlock=sps_lib/Electrical Machines/Synchronous Machine Control/Excitation System
  Hydraulic Turbine and Governor : spsHydraulicTurbineandGovernorLib/Hydraulic Turbine and Governor  sm="[ 10/3  0.07 ]"  gate="[  0.01  0.97518  -0.1  0.1 ]"  reg="[  0.05  1.163  0.105  0  0.01  ]"  hyd="[  0  2.67  ]"  dref=0  po=0.7516
      settings: LibrarySourceBlock=|
      | sps_lib/Electrical Machines/Synchronous Machine Control/Hydraulic Turbine
      | and Governor
  Stabilitator : Subsystem
  Terminator : Terminator
  wref : Constant
  wref1 : Constant
  Pm : Outport
  Vf : Outport  Port=2
  wires:
  pref/1 -> Hydraulic Turbine and Governor/2
  Complex to Real-Imag/2 -> Excitation System/3
  wref/1 -> Hydraulic Turbine and Governor/1
  Add/1 -> Stabilitator/3(dw), Hydraulic Turbine and Governor/5
  Vm/1 -> Complex to Real-Imag/1
  Pe 0/1 -> Stabilitator/2(Pe), Hydraulic Turbine and Governor/4
  Hydraulic Turbine and Governor/2 -> Terminator/1
  Stabilitator/1(Out1) -> Excitation System/4
  w/1 -> Add/1, Hydraulic Turbine and Governor/3
  Excitation System/1 -> Vf/1
  Hydraulic Turbine and Governor/1 -> Pm/1, Stabilitator/1(Pm)
  Vref/1 -> Excitation System/1
  wref1/1 -> Add/2
  Complex to Real-Imag/1 -> Excitation System/2

== system 43_BusNetworkElectricityTransmissionModel/South Network/Regulators 3/Turbine and Excitation Regulators ==
  pref : Inport
  w : Inport  Port=2
  Pe 0 : Inport  Port=3
  Vref : Inport  Port=4
  Vm : Inport  Port=5
  Add : Sum  Inputs=+-
  Complex to Real-Imag : ComplexToRealImag
  Excitation System : spsExcitationSystemLib/Excitation System  tr=20e-3  reg=[ 300, 0.001 ]  exc=[ 1, 0 ]  tgr=[ 0, 0 ]  damp=[ 0.001, 0.1 ]  sat=[ 0, 0 ]  lim=[ -11.5, 11.5, 0 ]  v0="[1.0  1.28]"
      settings: LibrarySourceBlock=sps_lib/Electrical Machines/Synchronous Machine Control/Excitation System
  Hydraulic Turbine and Governor : spsHydraulicTurbineandGovernorLib/Hydraulic Turbine and Governor  sm="[ 10/3  0.07 ]"  gate="[  0.01  0.97518  -0.1  0.1 ]"  reg="[  0.05  1.163  0.105  0  0.01  ]"  hyd="[  0  2.67  ]"  dref=0  po=0.7516
      settings: LibrarySourceBlock=|
      | sps_lib/Electrical Machines/Synchronous Machine Control/Hydraulic Turbine
      | and Governor
  Stabilitator : Subsystem
  Terminator : Terminator
  wref : Constant
  wref1 : Constant
  Pm : Outport
  Vf : Outport  Port=2
  wires:
  pref/1 -> Hydraulic Turbine and Governor/2
  Complex to Real-Imag/2 -> Excitation System/3
  wref/1 -> Hydraulic Turbine and Governor/1
  Add/1 -> Stabilitator/3(dw), Hydraulic Turbine and Governor/5
  Vm/1 -> Complex to Real-Imag/1
  Pe 0/1 -> Stabilitator/2(Pe), Hydraulic Turbine and Governor/4
  Hydraulic Turbine and Governor/2 -> Terminator/1
  Stabilitator/1(Out1) -> Excitation System/4
  w/1 -> Add/1, Hydraulic Turbine and Governor/3
  Excitation System/1 -> Vf/1
  Hydraulic Turbine and Governor/1 -> Pm/1, Stabilitator/1(Pm)
  Vref/1 -> Excitation System/1
  wref1/1 -> Add/2
  Complex to Real-Imag/1 -> Excitation System/2

== system 43_BusNetworkElectricityTransmissionModel/South Network/Regulators 4/Turbine and Excitation Regulators ==
  pref : Inport
  w : Inport  Port=2
  Pe 0 : Inport  Port=3
  Vref : Inport  Port=4
  Vm : Inport  Port=5
  Add : Sum  Inputs=+-
  Complex to Real-Imag : ComplexToRealImag
  Excitation System : spsExcitationSystemLib/Excitation System  tr=20e-3  reg=[ 300, 0.001 ]  exc=[ 1, 0 ]  tgr=[ 0, 0 ]  damp=[ 0.001, 0.1 ]  sat=[ 0, 0 ]  lim=[ -11.5, 11.5, 0 ]  v0="[1.0  1.28]"
      settings: LibrarySourceBlock=sps_lib/Electrical Machines/Synchronous Machine Control/Excitation System
  Hydraulic Turbine and Governor : spsHydraulicTurbineandGovernorLib/Hydraulic Turbine and Governor  sm="[ 10/3  0.07 ]"  gate="[  0.01  0.97518  -0.1  0.1 ]"  reg="[  0.05  1.163  0.105  0  0.01  ]"  hyd="[  0  2.67  ]"  dref=0  po=0.7516
      settings: LibrarySourceBlock=|
      | sps_lib/Electrical Machines/Synchronous Machine Control/Hydraulic Turbine
      | and Governor
  Stabilitator : Subsystem
  Terminator : Terminator
  wref : Constant
  wref1 : Constant
  Pm : Outport
  Vf : Outport  Port=2
  wires:
  pref/1 -> Hydraulic Turbine and Governor/2
  Complex to Real-Imag/2 -> Excitation System/3
  wref/1 -> Hydraulic Turbine and Governor/1
  Add/1 -> Hydraulic Turbine and Governor/5, Stabilitator/3(dw)
  Vm/1 -> Complex to Real-Imag/1
  Pe 0/1 -> Stabilitator/2(Pe), Hydraulic Turbine and Governor/4
  Hydraulic Turbine and Governor/2 -> Terminator/1
  Stabilitator/1(Out1) -> Excitation System/4
  w/1 -> Add/1, Hydraulic Turbine and Governor/3
  Excitation System/1 -> Vf/1
  Hydraulic Turbine and Governor/1 -> Pm/1, Stabilitator/1(Pm)
  Vref/1 -> Excitation System/1
  wref1/1 -> Add/2
  Complex to Real-Imag/1 -> Excitation System/2

== system 43_BusNetworkElectricityTransmissionModel/South Network/Regulators 5/Turbine and Excitation Regulators ==
  pref : Inport
  w : Inport  Port=2
  Pe 0 : Inport  Port=3
  Vref : Inport  Port=4
  Vm : Inport  Port=5
  Add : Sum  Inputs=+-
  Complex to Real-Imag : ComplexToRealImag
  Excitation System : spsExcitationSystemLib/Excitation System  tr=20e-3  reg=[ 300, 0.001 ]  exc=[ 1, 0 ]  tgr=[ 0, 0 ]  damp=[ 0.001, 0.1 ]  sat=[ 0, 0 ]  lim=[ -11.5, 11.5, 0 ]  v0="[1.0  1.28]"
      settings: LibrarySourceBlock=sps_lib/Electrical Machines/Synchronous Machine Control/Excitation System
  Hydraulic Turbine and Governor : spsHydraulicTurbineandGovernorLib/Hydraulic Turbine and Governor  sm="[ 10/3  0.07 ]"  gate="[  0.01  0.97518  -0.1  0.1 ]"  reg="[  0.05  1.163  0.105  0  0.01  ]"  hyd="[  0  2.67  ]"  dref=0  po=0.7516
      settings: LibrarySourceBlock=|
      | sps_lib/Electrical Machines/Synchronous Machine Control/Hydraulic Turbine
      | and Governor
  Stabilitator : Subsystem
  Terminator : Terminator
  wref : Constant
  wref1 : Constant
  Pm : Outport
  Vf : Outport  Port=2
  wires:
  pref/1 -> Hydraulic Turbine and Governor/2
  Complex to Real-Imag/2 -> Excitation System/3
  wref/1 -> Hydraulic Turbine and Governor/1
  Add/1 -> Stabilitator/3(dw), Hydraulic Turbine and Governor/5
  Vm/1 -> Complex to Real-Imag/1
  Pe 0/1 -> Stabilitator/2(Pe), Hydraulic Turbine and Governor/4
  Hydraulic Turbine and Governor/2 -> Terminator/1
  Stabilitator/1(Out1) -> Excitation System/4
  w/1 -> Add/1, Hydraulic Turbine and Governor/3
  Excitation System/1 -> Vf/1
  Hydraulic Turbine and Governor/1 -> Pm/1, Stabilitator/1(Pm)
  Vref/1 -> Excitation System/1
  wref1/1 -> Add/2
  Complex to Real-Imag/1 -> Excitation System/2

== system 43_BusNetworkElectricityTransmissionModel/South Network/Regulators 6/Turbine and Excitation Regulators ==
  pref : Inport
  w : Inport  Port=2
  Pe 0 : Inport  Port=3
  Vref : Inport  Port=4
  Vm : Inport  Port=5
  Add : Sum  Inputs=+-
  Complex to Real-Imag : ComplexToRealImag
  Excitation System : spsExcitationSystemLib/Excitation System  tr=20e-3  reg=[ 300, 0.001 ]  exc=[ 1, 0 ]  tgr=[ 0, 0 ]  damp=[ 0.001, 0.1 ]  sat=[ 0, 0 ]  lim=[ -11.5, 11.5, 0 ]  v0="[1.0  1.28]"
      settings: LibrarySourceBlock=sps_lib/Electrical Machines/Synchronous Machine Control/Excitation System
  Hydraulic Turbine and Governor : spsHydraulicTurbineandGovernorLib/Hydraulic Turbine and Governor  sm="[ 10/3  0.07 ]"  gate="[  0.01  0.97518  -0.1  0.1 ]"  reg="[  0.05  1.163  0.105  0  0.01  ]"  hyd="[  0  2.67  ]"  dref=0  po=0.7516
      settings: LibrarySourceBlock=|
      | sps_lib/Electrical Machines/Synchronous Machine Control/Hydraulic Turbine
      | and Governor
  Stabilitator : Subsystem
  Terminator : Terminator
  wref : Constant
  wref1 : Constant
  Pm : Outport
  Vf : Outport  Port=2
  wires:
  pref/1 -> Hydraulic Turbine and Governor/2
  Complex to Real-Imag/2 -> Excitation System/3
  wref/1 -> Hydraulic Turbine and Governor/1
  Add/1 -> Stabilitator/3(dw), Hydraulic Turbine and Governor/5
  Vm/1 -> Complex to Real-Imag/1
  Pe 0/1 -> Stabilitator/2(Pe), Hydraulic Turbine and Governor/4
  Hydraulic Turbine and Governor/2 -> Terminator/1
  Stabilitator/1(Out1) -> Excitation System/4
  w/1 -> Add/1, Hydraulic Turbine and Governor/3
  Excitation System/1 -> Vf/1
  Hydraulic Turbine and Governor/1 -> Pm/1, Stabilitator/1(Pm)
  Vref/1 -> Excitation System/1
  wref1/1 -> Add/2
  Complex to Real-Imag/1 -> Excitation System/2

== system 43_BusNetworkElectricityTransmissionModel/ 41.4 MW Wind Generation/41.4 MW Wind Farm/10.35 MW Wind Turbine 1/Wind Turbine & Generator 1 ==
  Generator speed (pu) : Inport
  Constant : Constant  Value=14
  Shaft : Subsystem
  Turbine : Subsystem
  "Wind Turbine " : Subsystem  mask{WT_Coeff8=WT_Coeff, WT_Param=WT_Param, vw0=11, Pmech_Out=1.035e7, Ts=Ts}
      mask prompts: WT_Coeff8 "Wind Turbine Coefficients"; WT_Param "Wind Turbine Coefficients"; vw0 "Initial Wind Speed (m/s)"; Pmech_Out "Nominal Mechanical Output Power"; Ts "Sample Time"
  T_shaft (pu) : Outport  VectorParamsAs1DForOutWhenUnconnected=off
  wires:
  [Pitch_WT1] -> "Wind Turbine "/2(Pitch angle (deg))
  Shaft/1(T_shaft (pu)) -> T_shaft (pu)/1, Turbine/2(T_shaft (pu))
  Generator speed (pu)/1 -> Turbine/3(Generator speed (pu))
  Turbine/2(W_wt (pu)) -> "Wind Turbine "/1(Generator speed (pu)1)
  Turbine/1(Turbine speed) -> Shaft/1(Speed)
  Constant/1 -> "Wind Turbine "/3(Wind speed (m/s))
  "Wind Turbine "/1(Tt (pu)) -> Turbine/1(T_wt (pu))

== system 43_BusNetworkElectricityTransmissionModel/ 41.4 MW Wind Generation/41.4 MW Wind Farm/10.35 MW Wind Turbine 2/Wind Turbine & Generator 1 ==
  Generator speed (pu) : Inport
  Constant : Constant  Value=14
  Shaft : Subsystem
  Turbine : Subsystem
  "Wind Turbine " : Subsystem  mask{WT_Coeff8=WT_Coeff, WT_Param=WT_Param, vw0=11, Pmech_Out=1.035e7, Ts=Ts}
      mask prompts: WT_Coeff8 "Wind Turbine Coefficients"; WT_Param "Wind Turbine Coefficients"; vw0 "Initial Wind Speed (m/s)"; Pmech_Out "Nominal Mechanical Output Power"; Ts "Sample Time"
  T_shaft (pu) : Outport  VectorParamsAs1DForOutWhenUnconnected=off
  wires:
  [Pitch_WT1] -> "Wind Turbine "/2(Pitch angle (deg))
  Shaft/1(T_shaft (pu)) -> T_shaft (pu)/1, Turbine/2(T_shaft (pu))
  Generator speed (pu)/1 -> Turbine/3(Generator speed (pu))
  Turbine/2(W_wt (pu)) -> "Wind Turbine "/1(Generator speed (pu)1)
  Turbine/1(Turbine speed) -> Shaft/1(Speed)
  Constant/1 -> "Wind Turbine "/3(Wind speed (m/s))
  "Wind Turbine "/1(Tt (pu)) -> Turbine/1(T_wt (pu))

== system 43_BusNetworkElectricityTransmissionModel/ 41.4 MW Wind Generation/41.4 MW Wind Farm/10.35 MW Wind Turbine 3/Wind Turbine & Generator 1 ==
  Generator speed (pu) : Inport
  Constant : Constant  Value=14
  Shaft : Subsystem
  Turbine : Subsystem
  "Wind Turbine " : Subsystem  mask{WT_Coeff8=WT_Coeff, WT_Param=WT_Param, vw0=11, Pmech_Out=1.035e7, Ts=Ts}
      mask prompts: WT_Coeff8 "Wind Turbine Coefficients"; WT_Param "Wind Turbine Coefficients"; vw0 "Initial Wind Speed (m/s)"; Pmech_Out "Nominal Mechanical Output Power"; Ts "Sample Time"
  T_shaft (pu) : Outport  VectorParamsAs1DForOutWhenUnconnected=off
  wires:
  [Pitch_WT1] -> "Wind Turbine "/2(Pitch angle (deg))
  Shaft/1(T_shaft (pu)) -> T_shaft (pu)/1, Turbine/2(T_shaft (pu))
  Generator speed (pu)/1 -> Turbine/3(Generator speed (pu))
  Turbine/2(W_wt (pu)) -> "Wind Turbine "/1(Generator speed (pu)1)
  Turbine/1(Turbine speed) -> Shaft/1(Speed)
  Constant/1 -> "Wind Turbine "/3(Wind speed (m/s))
  "Wind Turbine "/1(Tt (pu)) -> Turbine/1(T_wt (pu))

== system 43_BusNetworkElectricityTransmissionModel/ 41.4 MW Wind Generation/41.4 MW Wind Farm/10.35 MW Wind Turbine 4/Wind Turbine & Generator 1 ==
  Generator speed (pu) : Inport
  Constant : Constant  Value=14
  Shaft : Subsystem
  Turbine : Subsystem
  "Wind Turbine " : Subsystem  mask{WT_Coeff8=WT_Coeff, WT_Param=WT_Param, vw0=11, Pmech_Out=1.035e7, Ts=Ts}
      mask prompts: WT_Coeff8 "Wind Turbine Coefficients"; WT_Param "Wind Turbine Coefficients"; vw0 "Initial Wind Speed (m/s)"; Pmech_Out "Nominal Mechanical Output Power"; Ts "Sample Time"
  T_shaft (pu) : Outport  VectorParamsAs1DForOutWhenUnconnected=off
  wires:
  [Pitch_WT1] -> "Wind Turbine "/2(Pitch angle (deg))
  Shaft/1(T_shaft (pu)) -> T_shaft (pu)/1, Turbine/2(T_shaft (pu))
  Generator speed (pu)/1 -> Turbine/3(Generator speed (pu))
  Turbine/2(W_wt (pu)) -> "Wind Turbine "/1(Generator speed (pu)1)
  Turbine/1(Turbine speed) -> Shaft/1(Speed)
  Constant/1 -> "Wind Turbine "/3(Wind speed (m/s))
  "Wind Turbine "/1(Tt (pu)) -> Turbine/1(T_wt (pu))

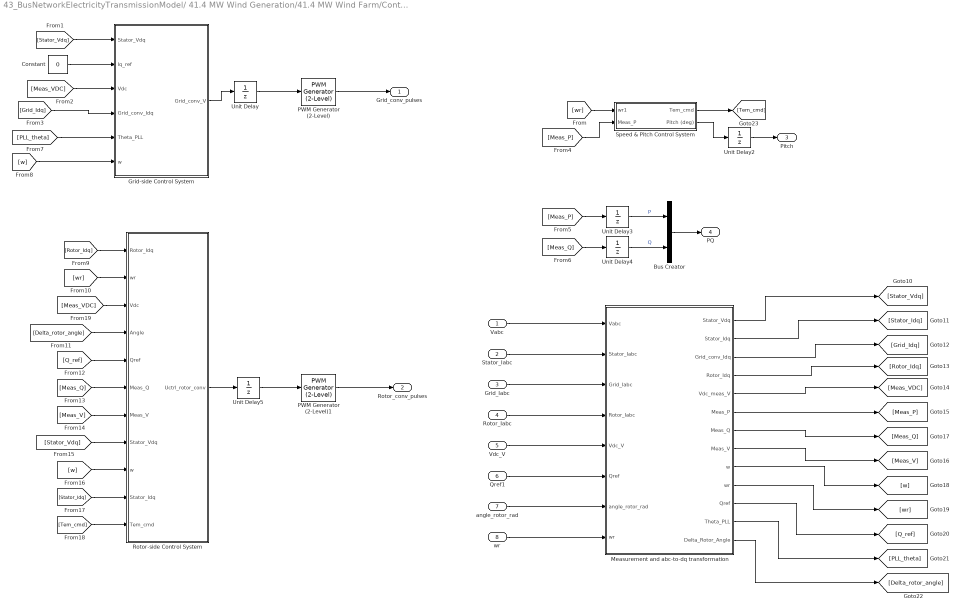
== system 43_BusNetworkElectricityTransmissionModel/ 41.4 MW Wind Generation/41.4 MW Wind Farm/Control System/Control System 1 ==
  Vabc : Inport
  Stator_Iabc : Inport  Port=2
  Grid_Iabc : Inport  Port=3
  Rotor_Iabc : Inport  Port=4
  Vdc_V : Inport  Port=5
  Qref1 : Inport  Port=6
  angle_rotor_rad : Inport  Port=7
  wr : Inport  Port=8
  Bus Creator : BusCreator  Inputs=P,Q
  Constant : Constant  Value=0
  Grid-side Control System : Subsystem
  "Measurement and abc-to-dq transformation " : Subsystem
  PWM Generator (2-Level) : spsPWMGenerator2LevelLib/PWM Generator (2-Level)  ModulatorType=Three-phase bridge (6 pulses)  ModulatorMode=Unsynchronized  Fc=Grid_Freq_PWM  Pc=90  nF=27  MinMax="[ -1  1 ]"  SamplingTechnique=Natural  ModulatingSignals=off  m=0.8  Freq=60  Phase=0  Ts=Ts  ShowCarrierOutport=off
  PWM Generator (2-Level)1 : spsPWMGenerator2LevelLib/PWM Generator (2-Level)  ModulatorType=Three-phase bridge (6 pulses)  ModulatorMode=Unsynchronized  Fc=Rotor_Freq_PWM  Pc=90  nF=27  MinMax="[ -1  1 ]"  SamplingTechnique=Natural  ModulatingSignals=off  m=0.8  Freq=60  Phase=0  Ts=Ts  ShowCarrierOutport=off
  Rotor-side Control System : Subsystem
  Speed & Pitch Control System : Subsystem
  Unit Delay{,2..5} (5 alike) : UnitDelay  SampleTime=Ts  HasFrameUpgradeWarning=on
  Grid_conv_pulses : Outport
  Rotor_conv_pulses : Outport  Port=2
  Pitch : Outport  Port=3
  PQ : Outport  Port=4
  wires:
  [Meas_P] -> Speed & Pitch Control System/2(Meas_P)
  "Measurement and abc-to-dq transformation "/1(Stator_Vdq) -> [Stator_Vdq]
  [Meas_Q] -> Unit Delay4/1
  Unit Delay4/1 -> Bus Creator/2  "Q"
  "Measurement and abc-to-dq transformation "/2(Stator_Idq) -> [Stator_Idq]
  "Measurement and abc-to-dq transformation "/9(w) -> [w]
  Grid_Iabc/1 -> "Measurement and abc-to-dq transformation "/3(Grid_Iabc)
  Grid-side Control System/1(Grid_conv_V) -> Unit Delay/1
  Unit Delay5/1 -> PWM Generator (2-Level)1/1
  Unit Delay2/1 -> Pitch/1
  Unit Delay/1 -> PWM Generator (2-Level)/1
  "Measurement and abc-to-dq transformation "/3(Grid_conv_Idq) -> [Grid_Idq]
  Rotor-side Control System/1(Uctrl_rotor_conv) -> Unit Delay5/1
  "Measurement and abc-to-dq transformation "/13(Delta_Rotor_Angle) -> [Delta_rotor_angle]
  PWM Generator (2-Level)/1 -> Grid_conv_pulses/1
  Vabc/1 -> "Measurement and abc-to-dq transformation "/1(Vabc)
  PWM Generator (2-Level)1/1 -> Rotor_conv_pulses/1
  "Measurement and abc-to-dq transformation "/4(Rotor_Idq) -> [Rotor_Idq]
  "Measurement and abc-to-dq transformation "/5(Vdc_meas_V) -> [Meas_VDC]
  angle_rotor_rad/1 -> "Measurement and abc-to-dq transformation "/7(angle_rotor_rad)
  wr/1 -> "Measurement and abc-to-dq transformation "/8(wr)
  "Measurement and abc-to-dq transformation "/7(Meas_Q) -> [Meas_Q]
  Speed & Pitch Control System/2(Pitch (deg)) -> Unit Delay2/1
  Stator_Iabc/1 -> "Measurement and abc-to-dq transformation "/2(Stator_Iabc)
  Speed & Pitch Control System/1(Tem_cmd) -> [Tem_cmd]
  Rotor_Iabc/1 -> "Measurement and abc-to-dq transformation "/4(Rotor_Iabc)
  Vdc_V/1 -> "Measurement and abc-to-dq transformation "/5(Vdc_V)
  Qref1/1 -> "Measurement and abc-to-dq transformation "/6(Qref)
  [wr] -> Speed & Pitch Control System/1(wr1)
  [Meas_P] -> Unit Delay3/1
  Unit Delay3/1 -> Bus Creator/1  "P"
  "Measurement and abc-to-dq transformation "/11("Qref ") -> [Q_ref]
  "Measurement and abc-to-dq transformation "/6(Meas_P) -> [Meas_P]
  "Measurement and abc-to-dq transformation "/12(Theta_PLL) -> [PLL_theta]
  Bus Creator/1 -> PQ/1
  "Measurement and abc-to-dq transformation "/8(Meas_V) -> [Meas_V]
  "Measurement and abc-to-dq transformation "/10("wr ") -> [wr]
  [Stator_Vdq] -> Grid-side Control System/1(Stator_Vdq)
  Constant/1 -> Grid-side Control System/2(Iq_ref)
  [Meas_VDC] -> Grid-side Control System/3(Vdc)
  [Grid_Idq] -> Grid-side Control System/4(Grid_conv_Idq)
  [PLL_theta] -> Grid-side Control System/5(Theta_PLL)
  [w] -> Grid-side Control System/6(w)
  [Rotor_Idq] -> Rotor-side Control System/1(Rotor_Idq)
  [wr] -> Rotor-side Control System/2(wr)
  [Meas_VDC] -> Rotor-side Control System/3(Vdc)
  [Delta_rotor_angle] -> Rotor-side Control System/4(Angle)
  [Q_ref] -> Rotor-side Control System/5(Qref)
  [Meas_Q] -> Rotor-side Control System/6(Meas_Q)
  [Meas_V] -> Rotor-side Control System/7(Meas_V)
  [Stator_Vdq] -> Rotor-side Control System/8(Stator_Vdq)
  [w] -> Rotor-side Control System/9(w)
  [Stator_Idq] -> Rotor-side Control System/10(Stator_Idq)
  [Tem_cmd] -> Rotor-side Control System/11(Tem_cmd)

== system 43_BusNetworkElectricityTransmissionModel/ 41.4 MW Wind Generation/41.4 MW Wind Farm/Control System/Control System 2 ==
  Vabc : Inport
  Stator_Iabc : Inport  Port=2
  Grid_Iabc : Inport  Port=3
  Rotor_Iabc : Inport  Port=4
  Vdc_V : Inport  Port=5
  Qref1 : Inport  Port=6
  angle_rotor_rad : Inport  Port=7
  wr : Inport  Port=8
  Bus Creator : BusCreator  Inputs=P,Q
  Constant : Constant  Value=0
  Grid-side Control System : Subsystem
  "Measurement and abc-to-dq transformation " : Subsystem
  PWM Generator (2-Level) : spsPWMGenerator2LevelLib/PWM Generator (2-Level)  ModulatorType=Three-phase bridge (6 pulses)  ModulatorMode=Unsynchronized  Fc=Grid_Freq_PWM  Pc=90  nF=27  MinMax="[ -1  1 ]"  SamplingTechnique=Natural  ModulatingSignals=off  m=0.8  Freq=60  Phase=0  Ts=Ts  ShowCarrierOutport=off
  PWM Generator (2-Level)1 : spsPWMGenerator2LevelLib/PWM Generator (2-Level)  ModulatorType=Three-phase bridge (6 pulses)  ModulatorMode=Unsynchronized  Fc=Rotor_Freq_PWM  Pc=90  nF=27  MinMax="[ -1  1 ]"  SamplingTechnique=Natural  ModulatingSignals=off  m=0.8  Freq=60  Phase=0  Ts=Ts  ShowCarrierOutport=off
  Rotor-side Control System : Subsystem
  Speed & Pitch Control System : Subsystem
  Unit Delay{,2..5} (5 alike) : UnitDelay  SampleTime=Ts  HasFrameUpgradeWarning=on
  Grid_conv_pulses : Outport
  Rotor_conv_pulses : Outport  Port=2
  Pitch : Outport  Port=3
  PQ : Outport  Port=4
  wires:
  [Meas_P] -> Speed & Pitch Control System/2(Meas_P)
  "Measurement and abc-to-dq transformation "/1(Stator_Vdq) -> [Stator_Vdq]
  [Meas_Q] -> Unit Delay4/1
  Unit Delay4/1 -> Bus Creator/2  "Q"
  "Measurement and abc-to-dq transformation "/2(Stator_Idq) -> [Stator_Idq]
  "Measurement and abc-to-dq transformation "/9(w) -> [w]
  Grid_Iabc/1 -> "Measurement and abc-to-dq transformation "/3(Grid_Iabc)
  Grid-side Control System/1(Grid_conv_V) -> Unit Delay/1
  Unit Delay5/1 -> PWM Generator (2-Level)1/1
  Unit Delay2/1 -> Pitch/1
  Unit Delay/1 -> PWM Generator (2-Level)/1
  "Measurement and abc-to-dq transformation "/3(Grid_conv_Idq) -> [Grid_Idq]
  Rotor-side Control System/1(Uctrl_rotor_conv) -> Unit Delay5/1
  "Measurement and abc-to-dq transformation "/13(Delta_Rotor_Angle) -> [Delta_rotor_angle]
  PWM Generator (2-Level)/1 -> Grid_conv_pulses/1
  Vabc/1 -> "Measurement and abc-to-dq transformation "/1(Vabc)
  PWM Generator (2-Level)1/1 -> Rotor_conv_pulses/1
  "Measurement and abc-to-dq transformation "/4(Rotor_Idq) -> [Rotor_Idq]
  "Measurement and abc-to-dq transformation "/5(Vdc_meas_V) -> [Meas_VDC]
  angle_rotor_rad/1 -> "Measurement and abc-to-dq transformation "/7(angle_rotor_rad)
  wr/1 -> "Measurement and abc-to-dq transformation "/8(wr)
  "Measurement and abc-to-dq transformation "/7(Meas_Q) -> [Meas_Q]
  Speed & Pitch Control System/2(Pitch (deg)) -> Unit Delay2/1
  Stator_Iabc/1 -> "Measurement and abc-to-dq transformation "/2(Stator_Iabc)
  Speed & Pitch Control System/1(Tem_cmd) -> [Tem_cmd]
  Rotor_Iabc/1 -> "Measurement and abc-to-dq transformation "/4(Rotor_Iabc)
  Vdc_V/1 -> "Measurement and abc-to-dq transformation "/5(Vdc_V)
  Qref1/1 -> "Measurement and abc-to-dq transformation "/6(Qref)
  [wr] -> Speed & Pitch Control System/1(wr1)
  [Meas_P] -> Unit Delay3/1
  Unit Delay3/1 -> Bus Creator/1  "P"
  "Measurement and abc-to-dq transformation "/11("Qref ") -> [Q_ref]
  "Measurement and abc-to-dq transformation "/6(Meas_P) -> [Meas_P]
  "Measurement and abc-to-dq transformation "/12(Theta_PLL) -> [PLL_theta]
  Bus Creator/1 -> PQ/1
  "Measurement and abc-to-dq transformation "/8(Meas_V) -> [Meas_V]
  "Measurement and abc-to-dq transformation "/10("wr ") -> [wr]
  [Stator_Vdq] -> Grid-side Control System/1(Stator_Vdq)
  Constant/1 -> Grid-side Control System/2(Iq_ref)
  [Meas_VDC] -> Grid-side Control System/3(Vdc)
  [Grid_Idq] -> Grid-side Control System/4(Grid_conv_Idq)
  [PLL_theta] -> Grid-side Control System/5(Theta_PLL)
  [w] -> Grid-side Control System/6(w)
  [Rotor_Idq] -> Rotor-side Control System/1(Rotor_Idq)
  [wr] -> Rotor-side Control System/2(wr)
  [Meas_VDC] -> Rotor-side Control System/3(Vdc)
  [Delta_rotor_angle] -> Rotor-side Control System/4(Angle)
  [Q_ref] -> Rotor-side Control System/5(Qref)
  [Meas_Q] -> Rotor-side Control System/6(Meas_Q)
  [Meas_V] -> Rotor-side Control System/7(Meas_V)
  [Stator_Vdq] -> Rotor-side Control System/8(Stator_Vdq)
  [w] -> Rotor-side Control System/9(w)
  [Stator_Idq] -> Rotor-side Control System/10(Stator_Idq)
  [Tem_cmd] -> Rotor-side Control System/11(Tem_cmd)
